simulink model "untitled"  (R2022b)
settings: Solver=ode23t  StartTime=0.0  StopTime=0.1  MaxStep=1e-5  RelTol=1e-3
undefined symbols (not defined in the file): C, Em, I_1_0, I_3_0, L, omega, R1, R2
libraries: fl_lib x8, nesl_utility x4
settings Model: Creator=hdu  LastModifiedBy=86156
settings ModelReferenceCC: EnableRefExpFcnMdlSchedulingChecks=on

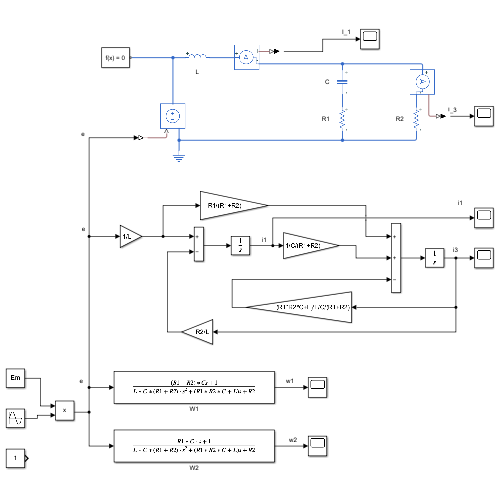
[thumbnail: Simulink's stored preview of the top-level diagram]
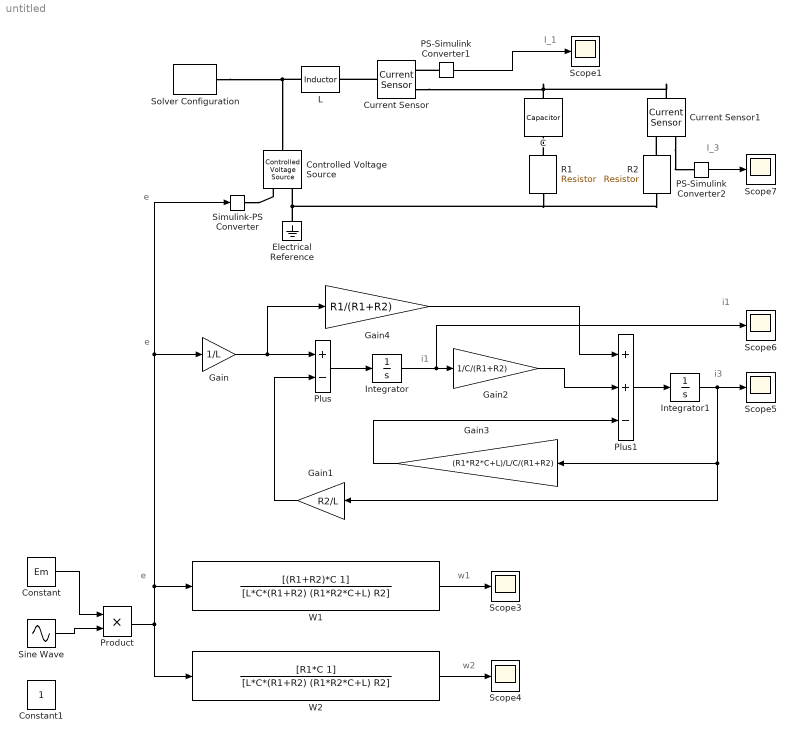
== system untitled ==
  note: e
  note: e
  note: e
  note: I_3
  note: w1
  note: i1
  note: i3
  note: i1
  note: I_1
  note: w2
  C : fl_lib/Electrical/Electrical Elements/Capacitor  c=C F  r=1e-6 Ohm  g=0 1/Ohm  i_specify=off  i_priority=None  i=0 A  i_nominal_specify=off  i_nominal_unit=A  i_nominal_value=1  v_specify=off  v_priority=None  v=0 V  v_nominal_specify=off  v_nominal_unit=V  v_nominal_value=1  vc_specify=off  vc_priority=High  vc=0 V  vc_nominal_specify=off  vc_nominal_unit=V  vc_nominal_value=1
  Constant : Constant  Value=Em
  Constant1 : Constant
  Controlled Voltage Source : fl_lib/Electrical/Electrical Sources/Controlled Voltage Source
  Current Sensor : fl_lib/Electrical/Electrical Sensors/Current Sensor
  Current Sensor1 : fl_lib/Electrical/Electrical Sensors/Current Sensor
  Electrical Reference : fl_lib/Electrical/Electrical Elements/Electrical Reference
  Gain : Gain  Gain=1/L
  Gain1 : Gain  Gain=R2/L
  Gain2 : Gain  Gain=1/C/(R1+R2)
  Gain3 : Gain  Gain=(R1*R2*C+L)/L/C/(R1+R2)
  Gain4 : Gain  Gain=R1/(R1+R2)
  Integrator : Integrator  InitialCondition=I_1_0*0
  Integrator1 : Integrator  InitialCondition=I_3_0*0
  L : fl_lib/Electrical/Electrical Elements/Inductor  l=L H  r=0 Ohm  g=1e-9 1/Ohm  i_specify=off  i_priority=None  i=0 A  i_nominal_specify=off  i_nominal_unit=A  i_nominal_value=1  v_specify=off  v_priority=None  v=0 V  v_nominal_specify=off  v_nominal_unit=V  v_nominal_value=1  i_L_specify=on  i_L_priority=High  i_L=I_1_0*0 A  i_L_nominal_specify=off  i_L_nominal_unit=A  i_L_nominal_value=1
  PS-Simulink Converter1 : nesl_utility/PS-Simulink Converter  PhysicalDomain=network_engine_domain  SubClassName=ps_output  LeftPortType=input  RightPortType=output  PseudoPeriodic=off  Frequencies=[]  VectorFormat=inherit  Unit=inherit  AffineConversion=off
  PS-Simulink Converter2 : nesl_utility/PS-Simulink Converter  PhysicalDomain=network_engine_domain  SubClassName=ps_output  LeftPortType=input  RightPortType=output  PseudoPeriodic=off  Frequencies=[]  VectorFormat=inherit  Unit=inherit  AffineConversion=off
  Plus : Sum  Inputs=+-
  Plus1 : Sum  Inputs=++-
  Product : Product
  R1 : fl_lib/Electrical/Electrical Elements/Resistor  R=R1 Ohm  i_specify=off  i_priority=None  i=0 A  i_nominal_specify=off  i_nominal_unit=A  i_nominal_value=1  v_specify=off  v_priority=None  v=0 V  v_nominal_specify=off  v_nominal_unit=V  v_nominal_value=1
  R2 : fl_lib/Electrical/Electrical Elements/Resistor  R=R2 Ohm  i_specify=on  i_priority=None  i=I_3_0*0 A  i_nominal_specify=off  i_nominal_unit=A  i_nominal_value=1  v_specify=off  v_priority=None  v=0 V  v_nominal_specify=off  v_nominal_unit=V  v_nominal_value=1
  Scope{1,3..7} (6 alike) : Scope
  Simulink-PS Converter : nesl_utility/Simulink-PS Converter  PhysicalDomain=network_engine_domain  SubClassName=ps_input  LeftPortType=input  RightPortType=output  PseudoPeriodic=off  Frequencies=[]  NoiseDistribution=none  NoiseParameters=[]  Unit=1  AffineConversion=off  FilteringAndDerivatives=provide  SimscapeFilterOrder=1  InputFilterTimeConstant=0.001  UdotUserProvided=0
  Sine Wave : Sin  Frequency=omega  SampleTime=0
  Solver Configuration : nesl_utility/Solver Configuration  PhysicalDomain=network_engine_domain  SubClassName=solver  LeftPortType=input  RightPortType=generic  Tones=[]  Harmonics=[]  SimulateNoise=off  Profile=off  UseLocalSampling=off  EnableSwitchedLinearOptims=on  FrequencyDomain=off  UseCCode=off  RelTol=0.001  AbsTol=0.001  MinStep=1e-09  ToWorkspace=off  RevertToSquareIcSolve=off  NumHomotopyIterations=100  PhasorMode=off  PhasorModeNumHarmonics=1  ConsistencySolver=NEWTON_FTOL  IndexReductionMethod=DerivativeReplacement  DoDC=off  ResidualTolerance=1e-09  ConsistencyTolSource=GLOBAL  ConsistencyAbsTol=0.001  ConsistencyRelTol=0.001  ConsistencyTolFactor=0.001  UseLocalSolver=off  LocalSolverChoice=NE_BACKWARD_EULER_ADVANCER  ResolveIndetEquations=on  FunctionEvalNumThread=1  LocalSolverSampleTime=0.001  DoFixedCost=off  MaxNonlinIter=3  MaxModeIter=2  ComputeImpulses=off  ImpulseIterations=2  LinearAlgebra=auto  LinearAlgebraNumThread=0  EquationFormulation=NE_TIME_EF  DelaysMemoryBudget=1024  AutomaticFiltering=on  FilteringTimeConstant=0.001  PartitionStorageMethod=AS_NEEDED  PartitionMemoryBudget=1024  PartitionMethod=ROBUST
  W1 : TransferFcn  Numerator=[(R1+R2)*C 1]  Denominator=[L*C*(R1+R2) (R1*R2*C+L) R2]
  W2 : TransferFcn  Numerator=[R1*C 1]  Denominator=[L*C*(R1+R2) (R1*R2*C+L) R2]
  wires:
  Constant/1 -> Product/1
  PS-Simulink Converter1/1 -> Scope1/1
  Product/1 -> Simulink-PS Converter/1, Gain/1, W1/1, W2/1
  Gain1/1 -> Plus/2
  Plus/1 -> Integrator/1
  Integrator/1 -> Scope6/1, Gain2/1
  Gain2/1 -> Plus1/2
  Plus1/1 -> Integrator1/1
  Integrator1/1 -> Scope5/1, Gain1/1, Gain3/1
  Gain3/1 -> Plus1/3
  Gain4/1 -> Plus1/1
  Gain/1 -> Gain4/1, Plus/1
  W1/1 -> Scope3/1
  W2/1 -> Scope4/1
  PS-Simulink Converter2/1 -> Scope7/1
  Sine Wave/1 -> Product/2
  connections:
  Simulink-PS Converter/RConn1 -- Controlled Voltage Source/RConn1
  Electrical Reference/LConn1 -- R1/RConn1 -- R2/RConn1 -- Controlled Voltage Source/RConn2
  Solver Configuration/RConn1 -- L/LConn1 -- Controlled Voltage Source/LConn1
  C/LConn1 -- Current Sensor1/LConn1 -- Current Sensor/RConn2
  R1/LConn1 -- C/RConn1
  Current Sensor/LConn1 -- L/RConn1
  PS-Simulink Converter1/LConn1 -- Current Sensor/RConn1
  R2/LConn1 -- Current Sensor1/RConn2
  Current Sensor1/RConn1 -- PS-Simulink Converter2/LConn1
